simulink model "SPWM_Three_Phase_Two_Level_Inverter"  (R2022a)
settings: Solver=VariableStepAuto  StartTime=0.0  StopTime=0.1  RelTol=1e-3
libraries: spsSawtoothGeneratorLib x1
settings Model: Creator=nikos  LastModifiedBy=nikos

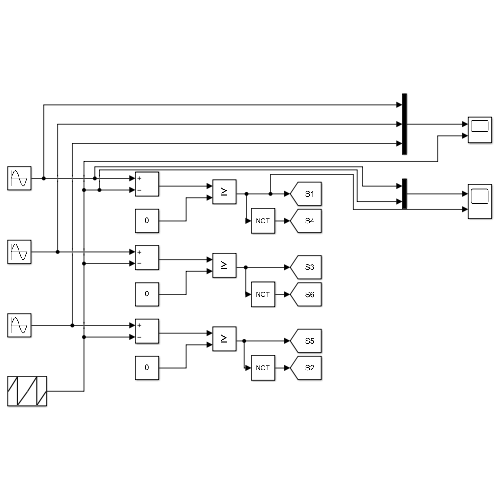
[thumbnail: Simulink's stored preview of the top-level diagram]
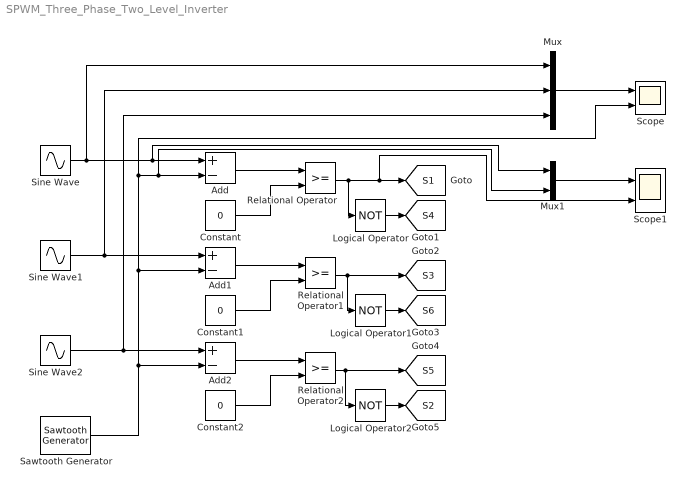
== system SPWM_Three_Phase_Two_Level_Inverter ==
  Add : Sum  Inputs=+-
  Add1 : Sum  Inputs=+-
  Add2 : Sum  Inputs=+-
  Constant : Constant  Value=0
  Constant1 : Constant  Value=0
  Constant2 : Constant  Value=0
  Logical Operator : Logic  Operator=NOT  AllPortsSameDT=off  OutDataTypeStr=boolean
  Logical Operator1 : Logic  Operator=NOT  AllPortsSameDT=off  OutDataTypeStr=boolean
  Logical Operator2 : Logic  Operator=NOT  AllPortsSameDT=off  OutDataTypeStr=boolean
  Mux : Mux  Inputs=3
  Mux1 : Mux  Inputs=2
  Relational Operator : RelationalOperator  OutDataTypeStr=boolean  RndMeth=Simplest  InputSameDT=off
  Relational Operator1 : RelationalOperator  OutDataTypeStr=boolean  RndMeth=Simplest  InputSameDT=off
  Relational Operator2 : RelationalOperator  OutDataTypeStr=boolean  RndMeth=Simplest  InputSameDT=off
  Sawtooth Generator : spsSawtoothGeneratorLib/Sawtooth Generator  Freq=1e3  Phase=180  Ts=0
  Scope : Scope  NumInputPorts=2
  Scope1 : Scope  NumInputPorts=2
  Sine Wave : Sin  Frequency=2*pi*50  SampleTime=0
  Sine Wave1 : Sin  Frequency=2*pi*50  Phase=4*pi/3  SampleTime=0
  Sine Wave2 : Sin  Frequency=2*pi*50  Phase=2*pi/3  SampleTime=0
  tag scope: S1=global, S2=global, S3=global, S4=global, S5=global, S6=global
  wires:
  Sine Wave/1 -> Add/1, Mux1/1, Mux/1
  Sine Wave1/1 -> Mux/2, Add1/1
  Sine Wave2/1 -> Mux/3, Add2/1
  Sawtooth Generator/1 -> Scope/2, Mux1/2, Add/2, Add1/2, Add2/2
  Add1/1 -> Relational Operator1/1
  Add/1 -> Relational Operator/1
  Constant/1 -> Relational Operator/2
  Add2/1 -> Relational Operator2/1
  Constant2/1 -> Relational Operator2/2
  Relational Operator/1 -> Logical Operator/1, Scope1/2, [S1]
  Logical Operator/1 -> [S4]
  Constant1/1 -> Relational Operator1/2
  Relational Operator1/1 -> Logical Operator1/1, [S3]
  Logical Operator1/1 -> [S6]
  Relational Operator2/1 -> Logical Operator2/1, [S5]
  Logical Operator2/1 -> [S2]
  Mux/1 -> Scope/1
  Mux1/1 -> Scope1/1
